simulink model "simulacion"  (R2021a)
settings: Solver=VariableStepAuto  StartTime=0.0  StopTime=10.0  RelTol=1e-3
undefined symbols (not defined in the file or in its folder): Gm
settings Model: Creator=pierr  LastModifiedBy=pierr

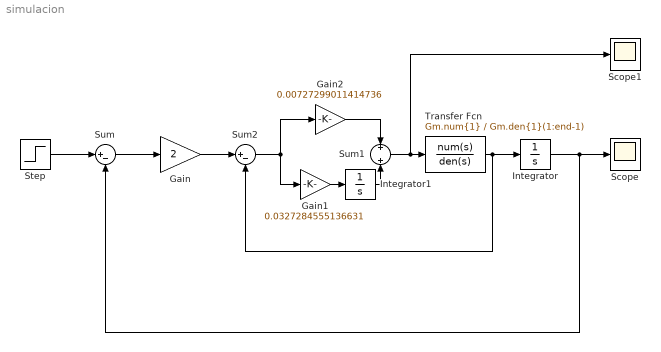
== system simulacion ==
  Gain : Gain  Gain=2
  Gain1 : Gain  Gain=0.0327284555136631
  Gain2 : Gain  Gain=0.00727299011414736
  Integrator : Integrator
  Integrator1 : Integrator
  Scope : Scope
  Scope1 : Scope
  Step : Step  Time=0  After=180  SampleTime=0
  Sum : Sum  Inputs=|+-
  Sum1 : Sum  Inputs=+||+
  Sum2 : Sum  Inputs=|+-
  Transfer Fcn : TransferFcn  Numerator=Gm.num{1}  Denominator=Gm.den{1}(1:end-1)
  wires:
  Sum/1 -> Gain/1
  Transfer Fcn/1 -> Sum2/2, Integrator/1
  Step/1 -> Sum/1
  Integrator/1 -> Scope/1, Sum/2
  Gain1/1 -> Integrator1/1
  Integrator1/1 -> Sum1/2
  Gain2/1 -> Sum1/1
  Gain/1 -> Sum2/1
  Sum2/1 -> Gain1/1, Gain2/1
  Sum1/1 -> Scope1/1, Transfer Fcn/1
